simulink model "simple_corr_audio_system_toolbox0x2810x29"  (R2024a)
settings: Solver=FixedStepDiscrete  StartTime=0.0  StopTime=0.55  RelTol=1e-3
PreLoadFcn:
  | load dspafxr;
libraries: dspstat3 x2, dspsrcs4 x1
settings Model: Creator=sv7  LastModifiedBy=zeqisun
settings SolverCC: AlgebraicLoopSolver=TrustRegion  PositivePriorityOrder=on
settings DataIOCC: SaveFormat=Array  SignalLoggingSaveFormat=ModelDataLogs  SaveOutput=off  SaveTime=off  ReturnWorkspaceOutputs=off
settings OptimizationCC: DefaultParameterBehavior=Inlined  InlineInvariantSignals=on  ExpressionDepthLimit=2147483647  InitFltsAndDblsToZero=on  LifeSpan=1
settings DebuggingCC: SaveWithParameterizedLinksMsg=none  UnderspecifiedInitializationDetection=Classic  MergeDetectMultiDrivingBlocksExec=none  SignalResolutionControl=TryResolveAllWithWarning  SolverPrmCheckMsg=warning  MultiTaskDSMMsg=warning  MultiTaskCondExecSysMsg=none  FcnCallInpInsideContextMsg=warning  UnconnectedInputMsg=warning  UnconnectedOutputMsg=warning  UnconnectedLineMsg=warning  StateNameClashWarn=warning  SFUnexpectedBacktrackingDiag=warning  SFNoUnconditionalDefaultTransitionDiag=warning  ArithmeticOperatorsInVariantConditions=warning
settings HardwareCC: ProdBitPerLong=40  ProdBitPerPointer=32  ProdBitPerSizeT=32  ProdBitPerPtrDiffT=32  ProdLargestAtomicInteger=Integer  ProdLargestAtomicFloat=None  ProdWordSize=32  ProdHWDeviceType=Texas Instruments->C6000  TargetBitPerLong=40  TargetLargestAtomicInteger=Integer  TargetIntDivRoundTo=Zero  TargetEndianess=LittleEndian  TargetHWDeviceType=TI C6000
settings ModelReferenceCC: EnableRefExpFcnMdlSchedulingChecks=on  PropagateSignalLabelsOutOfModel=off
settings SFSimCC: SimUseLocalCustomCode=off  CustomCodeUndefinedFunction=UseInterfaceOnly
settings RTWCC: Description=IDE Link ERT  SystemTargetFile=idelink_ert.tlc  GenerateMakefile=off  TemplateMakefile=none  RTWUseLocalCustomCode=off  GPUComputeCapability=3.5
settings CodeAppCC: StateflowObjectComments=on
settings TargetCC: CompOptLevelCompliant=off  ConcurrentExecutionCompliant=on  CombineOutputUpdateFcns=on  MATLABClassNameForMDSCustomization=linkfoundation.pjtgenerator.IdelinkCustomization  GRTInterface=off  InstructionSetFMA=off  OptimizeReductions=off  LogToMDFFile=off
settings ConfigComp: CovMetricSettings=dw  CovSaveCumulativeToWorkspaceVar=on  CovSaveSingleToWorkspaceVar=on  CovExternalEMLEnable=off
settings TargetHardwareResources: Description=Target Hardware Resources Component

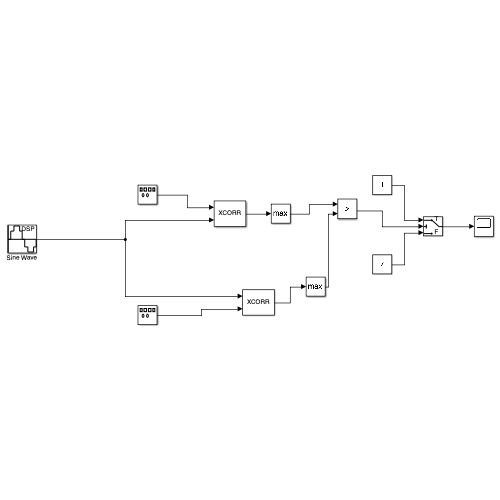
[thumbnail: Simulink's stored preview of the top-level diagram]
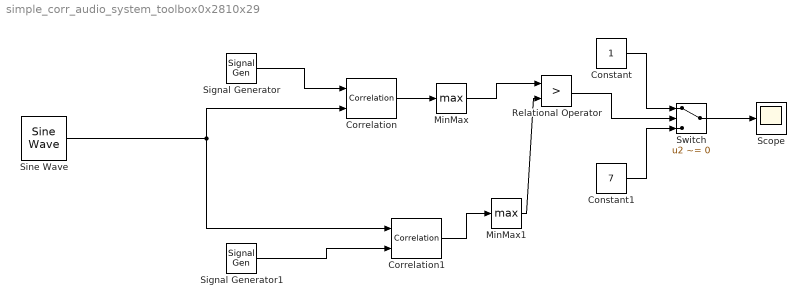
== system simple_corr_audio_system_toolbox0x2810x29 ==
  Constant : Constant
  Constant1 : Constant  Value=7
  Correlation : dspstat3/Correlation  domain=Time  roundingMode=Floor  overflowMode=off  outputDataTypeStr=Inherit: Same as accumulator  outputMin=[]  outputMax=[]  outputLastDataTypeStr=Inherit: Same as accumulator
  Correlation1 : dspstat3/Correlation  domain=Time  roundingMode=Floor  overflowMode=off  outputDataTypeStr=Inherit: Same as accumulator  outputMin=[]  outputMax=[]  outputLastDataTypeStr=Inherit: Same as accumulator
  MinMax : MinMax  Function=max
  MinMax1 : MinMax  Function=max
  Relational Operator : RelationalOperator  Operator=>  OutDataTypeStr=boolean  InputSameDT=off
  Scope : Scope
  Signal Generator : SignalGenerator  Frequency=697
  Signal Generator1 : SignalGenerator  Frequency=1477
  Sine Wave : dspsrcs4/Sine Wave  Amplitude=1  Frequency=1400  Phase=0  SampleMode=Discrete  OutComplex=Real  CompMethod=Trigonometric fcn  TableSize=Speed  SampleTime=1/8000  SamplesPerFrame=1  ResetState=Restart at time zero  OutputFrames=off  dataType=double  wordLen=16  udDataType=sfix(16)  fracBitsMode=Best precision  numFracBits=15  OutDataTypeStr=double  LastOutDataTypeStr=double
  Switch : Switch  Criteria=u2 ~= 0  SaturateOnIntegerOverflow=off  InputSameDT=off
  wires:
  Switch/1 -> Scope/1
  Relational Operator/1 -> Switch/2
  Constant1/1 -> Switch/3
  Constant/1 -> Switch/1
  Signal Generator1/1 -> Correlation1/2
  Signal Generator/1 -> Correlation/1
  Correlation/1 -> MinMax/1
  Correlation1/1 -> MinMax1/1
  MinMax1/1 -> Relational Operator/2
  MinMax/1 -> Relational Operator/1
  Sine Wave/1 -> Correlation/2, Correlation1/1
